simulink library "lib_discrete_time_integrator"  (R2023a)
settings: Solver=VariableStepAuto  StartTime=0.0  StopTime=10.0  RelTol=1e-3
undefined symbols (not defined in the file): cstMedTaskSampTime, cstSpdRampCoefMaxVal, dt_RpsElctSpd_s16p3b0
libraries: lib_conversion x7, lib_dynamic_saturator x2, lib_resettable_unit_delay x2
settings Model: Creator=cav2ofo  LastModifiedBy=xiaoqiang.yuan
settings OptimizationCC: ReuseModelBlockBuffer=off

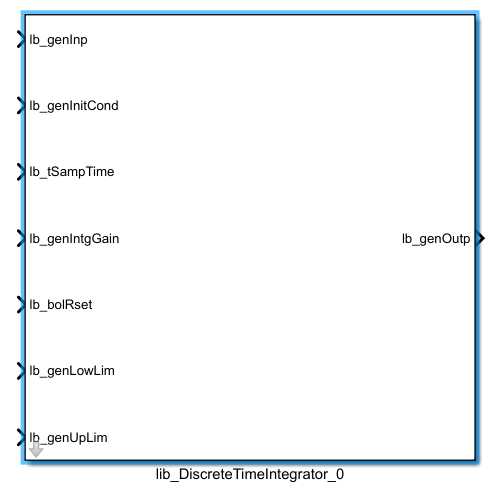
[thumbnail: Simulink's stored preview of the top-level diagram]
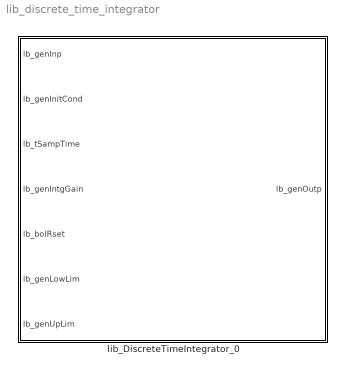
== system lib_discrete_time_integrator ==
  lib_DiscreteTimeIntegrator_0 : Subsystem  mask{lb_parMaxInpVal=cstSpdRampCoefMaxVal, lb_parMinInpVal=-cstSpdRampCoefMaxVal, lb_parMaxSampTime=double(cstMedTaskSampTime), lb_parMaxIntgGain=0, lb_parAccmDataTypeMode=32-bit, lb_parOutpDataType=dt_RpsElctSpd_s16p3b0, lb_parIntgScopMode=Generic signal, lb_parSatFlag=on}
      mask prompts: lb_parMaxInpVal "Maximum input value [iu]:"; lb_parMinInpVal "Minimum input value [iu]:"; lb_parMaxSampTime "Maximum sampling time [s]:"; lb_parMaxIntgGain "Maximum integral gain [ou/(iu*s)]:"; lb_parAccmDataTypeMode "Accumulator data type mode:"; lb_parOutpDataType "Output data type:"; lb_parIntgScopMode "Integration scope:"; lb_parSatFlag "Output saturation"
      mask init:
      | %% u is input signal
      | %% Ts is sampling time
      | %% Ki is integral gain
      | 
      | %% Convert to double parameters needed to compute data types
      | lb_parMaxInpVal = double(lb_parMaxInpVal);
      | lb_parMinInpVal = double(lb_parMinInpVal);
      | lb_parMaxSampTime = double(lb_parMaxSampTime);
      | lb_parMaxIntgGain = double(lb_parMaxIntgGain);
      | 
      | %% Req. XXX_030 - Define data type for integral loop
      | lb_parAccmDataType = Simulink.NumericType;
      | lb_parAccmDataType.DataTypeMode = 'Fixed-point: slope and bias scaling';
      | lb_parAccmDataType.Signedness = lb_parOutpDataType.Signedness;
      | switch lb_parAccmDataTypeMode
      |     case 'Same of output'
      |         lb_parAccmDataType.WordLength = lb_parOutpDataType.WordLength;
      |         lb_parAccmDataType.Slope = lb_parOutpDataType.Slope;
      |     case '32-bit'
      |         if lb_parOutpDataType.WordLength ~= 32
      |             lb_parAccmDataType.WordLength = 32;
      |             lb_parAccmDataType.Slope = lb_parOutpDataType.Slope*2^-16;
      |         else
      |             lb_parAccmDataType.WordLength = lb_parOutpDataType.WordLength;
      |             lb_parAccmDataType.Slope = lb_parOutpDataType.Slope;
      |         end
      | end
      | 
      | %% Req. XXX_031, 032, 033, 034 - Define of data type for product u*Ts
      | lb_parIntgStepDataTypeMaxVal = lb_parMaxInpVal*lb_parMaxSampTime;
      | lb_parIntgStepDataType = Simulink.NumericType;
      | lb_parIntgStepDataType.DataTypeMode= 'Fixed-point: unspecified scaling';
      | if lb_parMinInpVal < 0
      |     lb_parIntgStepDataType.Signedness = 'Signed';
      |     if lb_parIntgStepDataTypeMaxVal <= (2^16)/2-1 && lb_parAccmDataType.WordLength ~= 32
      |         lb_parIntgStepDataType.WordLength = 16;
      |     else
      |         lb_parIntgStepDataType.WordLength = 32;
      |     end
      | else
      |     lb_parIntgStepDataType.Signedness = 'Unsigned';
      |     if lb_parIntgStepDataTypeMaxVal <= (2^16)-1 && lb_parAccmDataType.WordLength ~= 32
      |         lb_parIntgStepDataType.WordLength = 16;
      |     else
      |         lb_parIntgStepDataType.WordLength = 32;
      |     end
      | end
      | 
      | %% Restore any suppressed diagnostics
      | Simulink.restoreDiagnostic(gcb);
      | 
      | %% Activate variant subsystem choice by means of set_param function
      | switch lb_parIntgScopMode
      |     
      |     case 'Generic signal'
      |         
      |         set_param([gcb,'/vss_IntegrationMode'],'LabelModeActiveChoice','lb_parGenSigModeLbl');
      |     
      |     case 'Angular signal'
      |         
      |         set_param([gcb,'/vss_IntegrationMode'],'LabelModeActiveChoice','lb_parGenSigModeLbl');
      |         
      |         %% Suppress diagnostics for sum block to avoid undesired warnings
      |         %  related to intentional overflow wrapping
      |         Simulink.suppressDiagnostic([gcb,'/vss_IntegrationMode/vss_GenericSignalMode/Sum'],...
      |             'SimulinkFixedPoint:util:Overflowoccurred');        
      |         
      |     case 'Integral control'
      |         
      |         %% Req. 035, 036, 037, 038 - Define a daty type for product u*Ts*Ki
      |         lb_parIntgCtrlDataTypeMaxVal = lb_parMaxIntgGain*lb_parIntgStepDataTypeMaxVal;
      |         lb_parIntgCtrlDataType = Simulink.NumericType;
      |         lb_parIntgCtrlDataType.DataTypeMode = 'Fixed-point: unspecified scaling';
      |         lb_parIntgCtrlDataType.Signedness = lb_parIntgStepDataType.Signedness;
      |         if lb_parMinInpVal < 0
      |             lb_parIntgCtrlDataType.Signedness = 'Signed';
      |             if lb_parIntgCtrlDataTypeMaxVal <= (2^16)/2-1 && lb_parAccmDataType.WordLength ~= 32
      |                 lb_parIntgCtrlDataType.WordLength = 16;
      |             else
      |                 lb_parIntgCtrlDataType.WordLength = 32;
      |             end
      |         else
      |             lb_parIntgCtrlDataType.Signedness = 'Unsigned';
      |             if lb_parIntgCtrlDataTypeMaxVal <= (2^16)-1 && lb_parAccmDataType.WordLength ~= 32
      |                 lb_parIntgCtrlDataType.WordLength = 16;
      |             else
      |                 lb_parIntgCtrlDataType.WordLength = 32;
      |             end
      |         end
      | 
      |         set_param([gcb,'/vss_IntegrationMode'],'LabelModeActiveChoice','lb_parIntgCtrlModeLbl');
      |         
      | end
      mask TypeOptions lb_parAccmDataTypeMode: Same of output | 32-bit
      mask TypeOptions lb_parIntgScopMode: Generic signal | Angular signal | Integral control
      mask DialogControl DescGroupVar Prompt: WEIFU motor control library
      mask DialogControl DescTextVar Prompt: Discrete time integrator
      mask DialogControl Container4 Prompt: Data types
      mask DialogControl Container3 Prompt: Operating modes

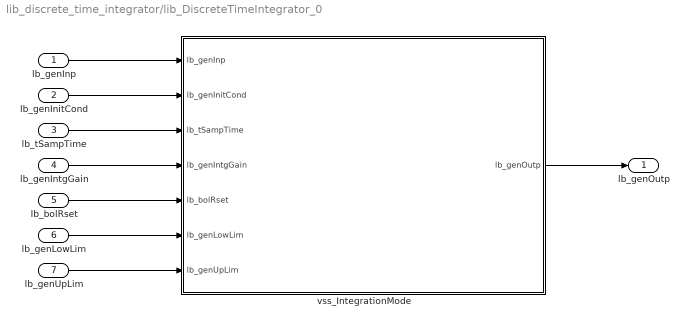
== system lib_discrete_time_integrator/lib_DiscreteTimeIntegrator_0 ==
  lb_genInp : Inport  OutMin=lb_parMinInpVal  OutMax=lb_parMaxInpVal
  lb_genInitCond : Inport  Port=2  OutDataTypeStr=lb_parOutpDataType
  lb_tSampTime : Inport  Port=3  OutMin=1e-9  OutMax=lb_parMaxSampTime
  lb_genIntgGain : Inport  Port=4  OutMin=0  OutMax=lb_parMaxIntgGain
  lb_bolRset : Inport  Port=5  OutDataTypeStr=boolean
  lb_genLowLim : Inport  Port=6  OutDataTypeStr=lb_parOutpDataType
  lb_genUpLim : Inport  Port=7  OutDataTypeStr=lb_parOutpDataType
  vss_IntegrationMode : Subsystem  Variant=on  VariantControlMode=label  LabelModeActiveChoice=lb_parGenSigModeLbl
  lb_genOutp : Outport
  wires:
  lb_genIntgGain/1 -> vss_IntegrationMode/4(lb_genIntgGain)
  lb_genInp/1 -> vss_IntegrationMode/1(lb_genInp)
  lb_genInitCond/1 -> vss_IntegrationMode/2(lb_genInitCond)
  lb_bolRset/1 -> vss_IntegrationMode/5(lb_bolRset)
  lb_genLowLim/1 -> vss_IntegrationMode/6(lb_genLowLim)
  lb_genUpLim/1 -> vss_IntegrationMode/7(lb_genUpLim)
  vss_IntegrationMode/1(lb_genOutp) -> lb_genOutp/1
  lb_tSampTime/1 -> vss_IntegrationMode/3(lb_tSampTime)

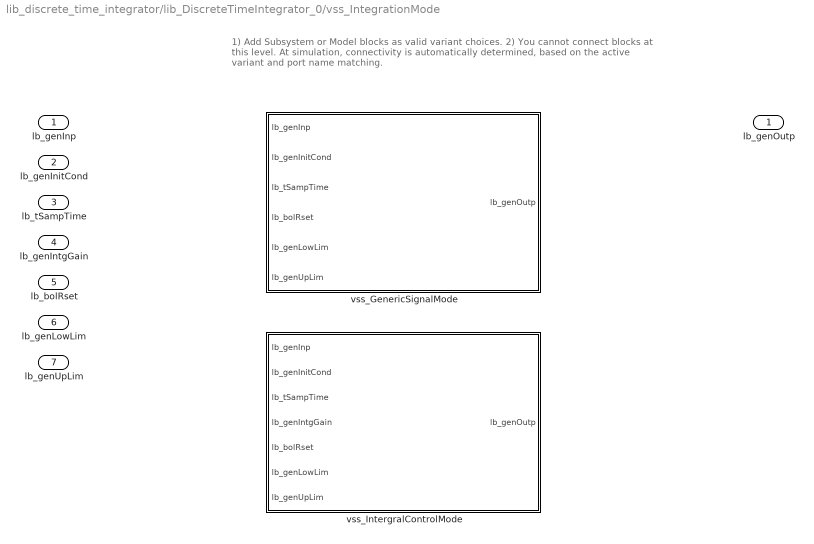
== system lib_discrete_time_integrator/lib_DiscreteTimeIntegrator_0/vss_IntegrationMode ==
  note: 1) Add Subsystem or Model blocks as valid variant choices.
      | 2) You cannot connect blocks at this level. At simulation, connectivity is automatically
      | determined, based on the active variant and port name matching.
  lb_genInp : Inport
  lb_genInitCond : Inport  Port=2
  lb_tSampTime : Inport  Port=3
  lb_genIntgGain : Inport  Port=4
  lb_bolRset : Inport  Port=5
  lb_genLowLim : Inport  Port=6
  lb_genUpLim : Inport  Port=7
  vss_GenericSignalMode : Subsystem  VariantControl=lb_parGenSigModeLbl
  vss_IntergralControlMode : Subsystem  VariantControl=lb_parIntgCtrlModeLbl
  lb_genOutp : Outport  VectorParamsAs1DForOutWhenUnconnected=off

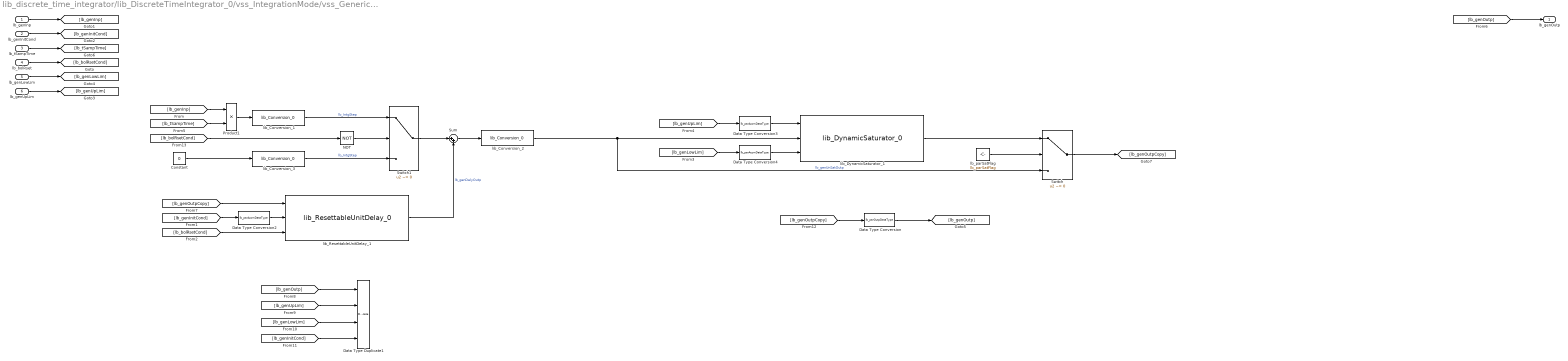
== system lib_discrete_time_integrator/lib_DiscreteTimeIntegrator_0/vss_IntegrationMode/vss_GenericSignalMode ==
  lb_genInp : Inport
  lb_genInitCond : Inport  Port=2
  lb_tSampTime : Inport  Port=3
  lb_bolRset : Inport  Port=4
  lb_genLowLim : Inport  Port=5
  lb_genUpLim : Inport  Port=6
  Constant : Constant  Value=0  OutDataTypeStr=Inherit: Inherit via back propagation
  Data Type Duplicate1 : DataTypeDuplicate  NumInputPorts=4
  Data Type Conversion : DataTypeConversion  OutDataTypeStr=lb_parOutpDataType  SaturateOnIntegerOverflow=off  RndMeth=Floor
  Data Type Conversion2 : DataTypeConversion  OutDataTypeStr=lb_parAccmDataType  SaturateOnIntegerOverflow=off  RndMeth=Floor
  Data Type Conversion3 : DataTypeConversion  OutDataTypeStr=lb_parAccmDataType  SaturateOnIntegerOverflow=off  RndMeth=Floor
  Data Type Conversion4 : DataTypeConversion  OutDataTypeStr=lb_parAccmDataType  SaturateOnIntegerOverflow=off  RndMeth=Floor
  NOT : Logic  Operator=NOT  AllPortsSameDT=off  OutDataTypeStr=boolean
  Product1 : Product  OutDataTypeStr=Inherit: Inherit via back propagation  RndMeth=Simplest
  Sum : Sum  Inputs=|++  OutDataTypeStr=Inherit: Inherit via back propagation  RndMeth=Simplest
  Switch : Switch  Criteria=u2 ~= 0  SaturateOnIntegerOverflow=off  InputSameDT=off
  Switch1 : Switch  Criteria=u2 ~= 0  SaturateOnIntegerOverflow=off  InputSameDT=off  OutDataTypeStr=Inherit: Same as first input
  lb_parSatFlag : Constant  Value=lb_parSatFlag  OutDataTypeStr=boolean
  lib_Conversion_1 : lib_conversion/lib_Conversion_0  lb_parDataType=lb_parIntgStepDataType  lb_parOutpMaxVal=lb_parIntgStepDataTypeMaxVal  lb_parOutpMinVal=[]  lb_parSatFlag=off
  lib_Conversion_2 : lib_conversion/lib_Conversion_0  lb_parDataType=lb_parAccmDataType  lb_parOutpMaxVal=[]  lb_parOutpMinVal=[]  lb_parSatFlag=off
  lib_Conversion_3 : lib_conversion/lib_Conversion_0  lb_parDataType=lb_parIntgStepDataType  lb_parOutpMaxVal=lb_parIntgStepDataTypeMaxVal  lb_parOutpMinVal=[]  lb_parSatFlag=off
  lib_DynamicSaturator_1 : lib_dynamic_saturator/lib_DynamicSaturator_0
  lib_ResettableUnitDelay_1 : lib_resettable_unit_delay/lib_ResettableUnitDelay_0
  lb_genOutp : Outport
  wires:
  lib_Conversion_3/1 -> Switch1/3  "lb_IntgStep"
  Constant/1 -> lib_Conversion_3/1
  Switch1/1 -> Sum/1
  NOT/1 -> Switch1/2
  [lb_bolRsetCond] -> NOT/1
  [lb_genUpLim] -> Data Type Conversion3/1
  Product1/1 -> lib_Conversion_1/1
  [lb_genOutp] -> lb_genOutp/1
  lb_tSampTime/1 -> [lb_tSampTime]
  lb_genInp/1 -> [lb_genInp]
  lb_parSatFlag/1 -> Switch/2
  lib_DynamicSaturator_1/1 -> Switch/1
  [lb_genLowLim] -> Data Type Conversion4/1
  lib_Conversion_2/1 -> lib_DynamicSaturator_1/2, Switch/3  "lb_genUnSatOutp"
  Data Type Conversion4/1 -> lib_DynamicSaturator_1/3
  Data Type Conversion/1 -> [lb_genOutp]
  [lb_tSampTime] -> Product1/2
  lib_Conversion_1/1 -> Switch1/1  "lb_IntgStep"
  Data Type Conversion3/1 -> lib_DynamicSaturator_1/1
  [lb_genInp] -> Product1/1
  lb_genUpLim/1 -> [lb_genUpLim]
  lb_genInitCond/1 -> [lb_genInitCond]
  lb_genLowLim/1 -> [lb_genLowLim]
  Sum/1 -> lib_Conversion_2/1
  lb_bolRset/1 -> [lb_bolRsetCond]
  [lb_genUpLim] -> Data Type Duplicate1/2
  [lb_genLowLim] -> Data Type Duplicate1/3
  [lb_genInitCond] -> Data Type Duplicate1/4
  [lb_genOutp] -> Data Type Duplicate1/1
  [lb_bolRsetCond] -> lib_ResettableUnitDelay_1/3
  Data Type Conversion2/1 -> lib_ResettableUnitDelay_1/2
  [lb_genInitCond] -> Data Type Conversion2/1
  lib_ResettableUnitDelay_1/1 -> Sum/2  "lb_genDelyOutp"
  Switch/1 -> [lb_genOutpCopy]
  [lb_genOutpCopy] -> lib_ResettableUnitDelay_1/1
  [lb_genOutpCopy] -> Data Type Conversion/1

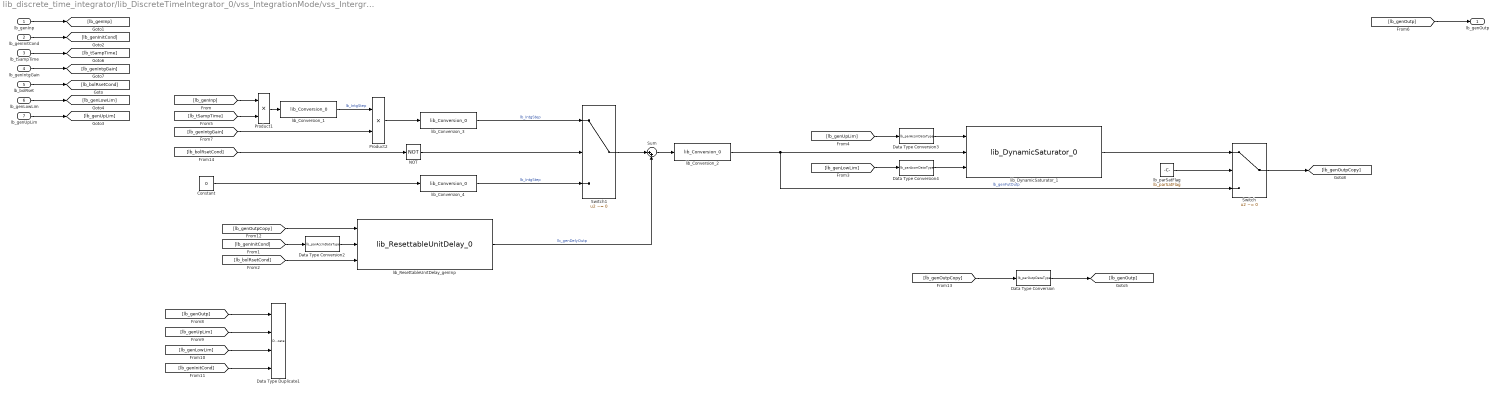
== system lib_discrete_time_integrator/lib_DiscreteTimeIntegrator_0/vss_IntegrationMode/vss_IntergralControlMode ==
  lb_genInp : Inport
  lb_genInitCond : Inport  Port=2
  lb_tSampTime : Inport  Port=3
  lb_genIntgGain : Inport  Port=4
  lb_bolRset : Inport  Port=5
  lb_genLowLim : Inport  Port=6
  lb_genUpLim : Inport  Port=7
  Constant : Constant  Value=0  OutDataTypeStr=Inherit: Inherit via back propagation
  Data Type Duplicate1 : DataTypeDuplicate  NumInputPorts=4
  Data Type Conversion : DataTypeConversion  OutDataTypeStr=lb_parOutpDataType  SaturateOnIntegerOverflow=off  RndMeth=Floor
  Data Type Conversion2 : DataTypeConversion  OutDataTypeStr=lb_parAccmDataType  SaturateOnIntegerOverflow=off  RndMeth=Floor
  Data Type Conversion3 : DataTypeConversion  OutDataTypeStr=lb_parAccmDataType  SaturateOnIntegerOverflow=off  RndMeth=Floor
  Data Type Conversion4 : DataTypeConversion  OutDataTypeStr=lb_parAccmDataType  SaturateOnIntegerOverflow=off  RndMeth=Floor
  NOT : Logic  Operator=NOT  AllPortsSameDT=off  OutDataTypeStr=boolean
  Product1 : Product  OutDataTypeStr=Inherit: Inherit via back propagation  RndMeth=Simplest
  Product2 : Product  OutDataTypeStr=Inherit: Inherit via back propagation  RndMeth=Simplest
  Sum : Sum  Inputs=|++  OutDataTypeStr=Inherit: Inherit via back propagation  RndMeth=Simplest
  Switch : Switch  Criteria=u2 ~= 0  SaturateOnIntegerOverflow=off  InputSameDT=off
  Switch1 : Switch  Criteria=u2 ~= 0  SaturateOnIntegerOverflow=off  InputSameDT=off  OutDataTypeStr=Inherit: Same as first input
  lb_parSatFlag : Constant  Value=lb_parSatFlag  OutDataTypeStr=boolean
  lib_Conversion_1 : lib_conversion/lib_Conversion_0  lb_parDataType=lb_parIntgStepDataType  lb_parOutpMaxVal=lb_parIntgStepDataTypeMaxVal  lb_parOutpMinVal=[]  lb_parSatFlag=off
  lib_Conversion_2 : lib_conversion/lib_Conversion_0  lb_parDataType=lb_parAccmDataType  lb_parOutpMaxVal=[]  lb_parOutpMinVal=[]  lb_parSatFlag=off
  lib_Conversion_3 : lib_conversion/lib_Conversion_0  lb_parDataType=lb_parIntgCtrlDataType  lb_parOutpMaxVal=lb_parIntgCtrlDataTypeMaxVal  lb_parOutpMinVal=[]  lb_parSatFlag=off
  lib_Conversion_4 : lib_conversion/lib_Conversion_0  lb_parDataType=lb_parIntgCtrlDataType  lb_parOutpMaxVal=lb_parIntgCtrlDataTypeMaxVal  lb_parOutpMinVal=[]  lb_parSatFlag=off
  lib_DynamicSaturator_1 : lib_dynamic_saturator/lib_DynamicSaturator_0
  lib_ResettableUnitDelay_genInp : lib_resettable_unit_delay/lib_ResettableUnitDelay_0
  lb_genOutp : Outport
  wires:
  Switch1/1 -> Sum/1
  NOT/1 -> Switch1/2
  [lb_bolRsetCond] -> NOT/1
  Constant/1 -> lib_Conversion_4/1
  lib_Conversion_3/1 -> Switch1/1  "lb_IntgStep"
  lib_Conversion_4/1 -> Switch1/3  "lb_IntgStep"
  Product2/1 -> lib_Conversion_3/1
  [lb_genUpLim] -> Data Type Conversion3/1
  Product1/1 -> lib_Conversion_1/1
  lib_Conversion_1/1 -> Product2/1  "lb_IntgStep"
  [lb_genOutp] -> lb_genOutp/1
  lb_tSampTime/1 -> [lb_tSampTime]
  lb_genInp/1 -> [lb_genInp]
  lb_parSatFlag/1 -> Switch/2
  lib_DynamicSaturator_1/1 -> Switch/1
  [lb_genLowLim] -> Data Type Conversion4/1
  Data Type Conversion2/1 -> lib_ResettableUnitDelay_genInp/2
  [lb_genInitCond] -> Data Type Conversion2/1
  Data Type Conversion4/1 -> lib_DynamicSaturator_1/3
  Data Type Conversion/1 -> [lb_genOutp]
  [lb_tSampTime] -> Product1/2
  Data Type Conversion3/1 -> lib_DynamicSaturator_1/1
  [lb_genInp] -> Product1/1
  lb_genUpLim/1 -> [lb_genUpLim]
  lb_genInitCond/1 -> [lb_genInitCond]
  [lb_bolRsetCond] -> lib_ResettableUnitDelay_genInp/3
  lb_genLowLim/1 -> [lb_genLowLim]
  lb_genIntgGain/1 -> [lb_genIntgGain]
  Sum/1 -> lib_Conversion_2/1
  lb_bolRset/1 -> [lb_bolRsetCond]
  [lb_genIntgGain] -> Product2/2
  [lb_genUpLim] -> Data Type Duplicate1/2
  [lb_genLowLim] -> Data Type Duplicate1/3
  [lb_genInitCond] -> Data Type Duplicate1/4
  [lb_genOutp] -> Data Type Duplicate1/1
  lib_Conversion_2/1 -> Switch/3, lib_DynamicSaturator_1/2  "lb_genFutOutp"
  [lb_genOutpCopy] -> lib_ResettableUnitDelay_genInp/1
  lib_ResettableUnitDelay_genInp/1 -> Sum/2  "lb_genDelyOutp"
  Switch/1 -> [lb_genOutpCopy]
  [lb_genOutpCopy] -> Data Type Conversion/1
